simulink model "bitcrusher"  (R2020b)
settings: Solver=FixedStepDiscrete  StartTime=0.0  StopTime=stopTime  RelTol=1e-3
InitFcn:
  | initCallback
StopFcn:
  | stopCallback
values from neighbouring files (symbols this model uses):
  mp = sm_init_avalon_signals(mp)    [sm_callback_init.m]
settings Model: Creator=Ross  LastModifiedBy=wickh
settings DataIOCC: ReturnWorkspaceOutputs=off
settings OptimizationCC: BlockReduction=off  ConditionallyExecuteInputs=off  DefaultParameterBehavior=Inlined
settings DebuggingCC: ReadBeforeWriteMsg=DisableAll  WriteAfterWriteMsg=DisableAll  WriteAfterReadMsg=DisableAll  AlgebraicLoopMsg=error  MultiTaskDSMMsg=none  SingleTaskRateTransMsg=error  PregeneratedLibrarySubsystemCodeDiagnostic=none  ArithmeticOperatorsInVariantConditions=warning
settings HardwareCC: ProdBitPerPointer=32  ProdBitPerSizeT=32  ProdBitPerPtrDiffT=32  ProdLargestAtomicFloat=None  ProdIntDivRoundTo=Undefined  ProdEndianess=Unspecified  ProdWordSize=32  ProdHWDeviceType=ASIC/FPGA->ASIC/FPGA  TargetBitPerPointer=64  TargetBitPerSizeT=64  TargetBitPerPtrDiffT=64  TargetLongLongMode=on  TargetIntDivRoundTo=Zero  TargetEndianess=LittleEndian  TargetWordSize=64  TargetHWDeviceType=Custom Processor->MATLAB Host Computer  ProdEqTarget=off
settings ModelReferenceCC: UpdateModelReferenceTargets=IfOutOfDate
settings SFSimCC: SFSimEcho=off  SimUseLocalCustomCode=off  CustomCodeUndefinedFunction=UseInterfaceOnly
settings RTWCC: RTWUseLocalCustomCode=off

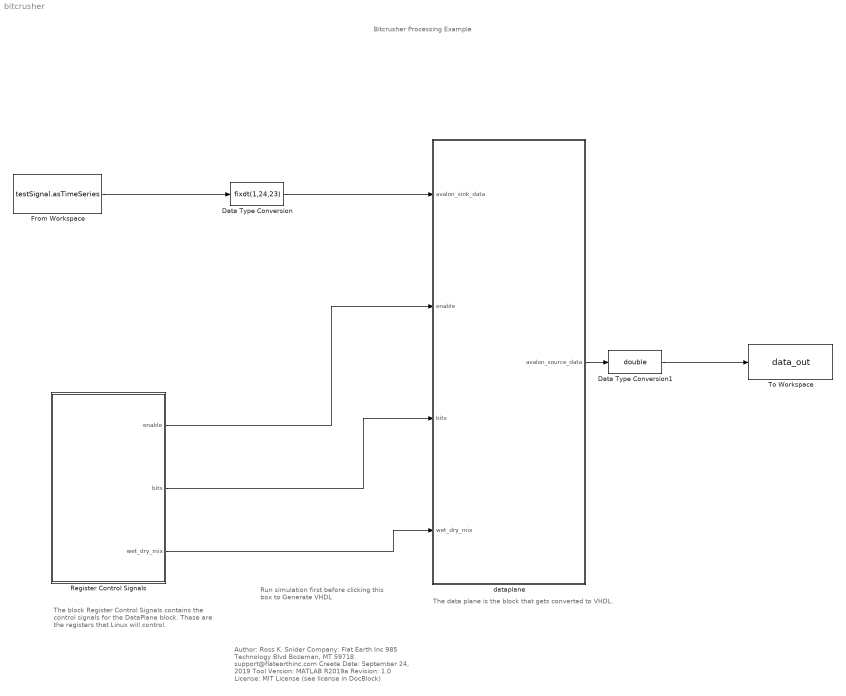
== system bitcrusher ==
  note: The data plane is the block that gets converted to VHDL.
  note: Author:          Ross K. Snider
      | Company:     Flat Earth Inc
      |                       985 Technology Blvd
      |                       Bozeman, MT 59718
      |                       support@flatearthinc.com
      | Create Date:  September 24, 2019
      | Tool Version:  MATLAB R2019a
      | Revision:        1.0
      | License:          MIT License (see license in DocBlock)
  note: Bitcrusher
      | Processing Example
  note: Run simulation first
      | before clicking this box to
      | Generate VHDL
  note: The block Register Control Signals contains
      | the control signals for the DataPlane block.
      | These are the registers that Linux will control.
  Data Type Conversion : DataTypeConversion  OutDataTypeStr=fixdt(1,24,23)
  Data Type Conversion1 : DataTypeConversion  OutDataTypeStr=double
  From Workspace : FromWorkspace  VariableName=testSignal.asTimeSeries  OutDataTypeStr=double  SampleTime=mp.Ts_sim  Interpolate=off  OutputAfterFinalValue=Setting to zero
  Register Control Signals : Subsystem
  To Workspace : ToWorkspace  VariableName=data_out  SampleTime=-1
  dataplane : Subsystem  TreatAsAtomicUnit=on
  wires:
  Data Type Conversion/1 -> dataplane/1(avalon_sink_data)
  Register Control Signals/2(bits) -> dataplane/3(bits)
  Register Control Signals/1(enable) -> dataplane/2(enable)
  Register Control Signals/3(wet_dry_mix) -> dataplane/4(wet_dry_mix)
  From Workspace/1 -> Data Type Conversion/1
  Data Type Conversion1/1 -> To Workspace/1
  dataplane/1(avalon_source_data) -> Data Type Conversion1/1

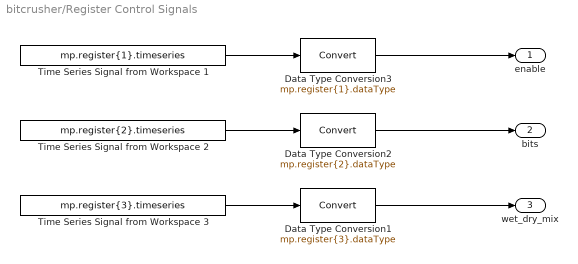
== system bitcrusher/Register Control Signals ==
  Data Type Conversion1 : DataTypeConversion  OutDataTypeStr=mp.register{3}.dataType
  Data Type Conversion2 : DataTypeConversion  OutDataTypeStr=mp.register{2}.dataType
  Data Type Conversion3 : DataTypeConversion  OutDataTypeStr=mp.register{1}.dataType
  Time Series Signal from Workspace 1 : FromWorkspace  VariableName=mp.register{1}.timeseries  OutDataTypeStr=double  SampleTime=mp.Ts_sim
  Time Series Signal from Workspace 2 : FromWorkspace  VariableName=mp.register{2}.timeseries  OutDataTypeStr=double  SampleTime=mp.Ts_sim
  Time Series Signal from Workspace 3 : FromWorkspace  VariableName=mp.register{3}.timeseries  OutDataTypeStr=double  SampleTime=mp.Ts_sim
  enable : Outport  VectorParamsAs1DForOutWhenUnconnected=off
  bits : Outport  Port=2  VectorParamsAs1DForOutWhenUnconnected=off
  wet_dry_mix : Outport  Port=3  VectorParamsAs1DForOutWhenUnconnected=off
  wires:
  Time Series Signal from Workspace 2/1 -> Data Type Conversion2/1
  Data Type Conversion2/1 -> bits/1
  Time Series Signal from Workspace 1/1 -> Data Type Conversion3/1
  Data Type Conversion3/1 -> enable/1
  Time Series Signal from Workspace 3/1 -> Data Type Conversion1/1
  Data Type Conversion1/1 -> wet_dry_mix/1

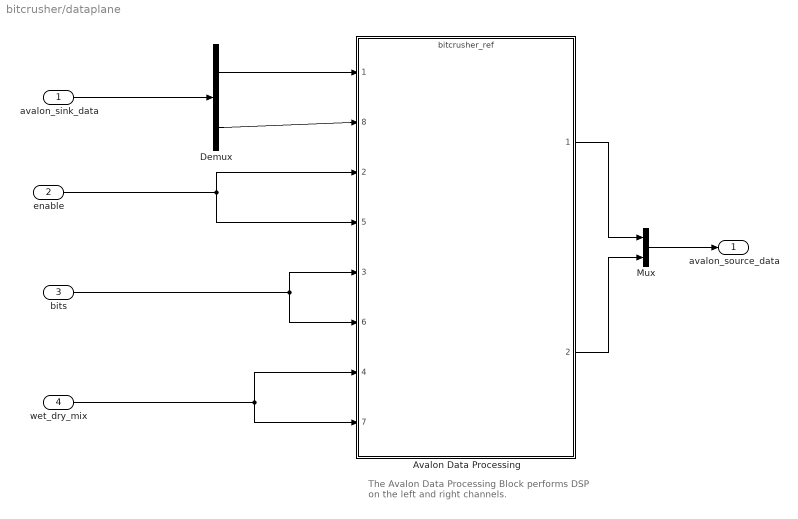
== system bitcrusher/dataplane ==
  note: The Avalon Data Processing Block
      | performs DSP on the left and right channels.
  avalon_sink_data : Inport
  enable : Inport  Port=2
  bits : Inport  Port=3
  wet_dry_mix : Inport  Port=4
  Avalon Data Processing : ModelReference  ModelNameDialog=bitcrusher_ref  SimulationMode=Normal  ModelReferenceVersion=3.10
      settings: PortSchema="{\"entries\":[{\"content\":{\"sides\":[{\"content\":{\"connectorIds\":[\"In1\",\"In8\",\"In2\",\"In5\",\"In3\",\"In6\",\"In4\",\"In7\"]},\"type\":\"ConnectorPlacement.EquallySpacedRectSide\",\"uuid\":\"cfc9476e-c101-4a90-ba08-effa479a8c46\"},{\"content\":{\"connectorIds\":[\"Out1\",\"Out2\"],\"side\":\"RIGHT\"},\"type\":\"ConnectorPlacement.EquallySpacedRectSide\",\"uuid\":\"4efa5dd5-d427-488d-bbaa-11ad48f52db2\"},{\"content\":{\"connectorIds\":[],\"side\":\"TOP\"},\"type\":\"ConnectorPlacement.EquallySpacedRectSide\",\"uuid\":\"d7e65a11-17aa-4e5c-94c4-a706f18cbe28\"},{\"content\":{\"connectorIds\":[],\"side\":\"HIDDEN\"},\"type\":\"ConnectorPlacement.EquallySpacedRectSide\",\"uuid\":\"578b30b2-4a86-4a40-9d9d-3e590ffd0d37\"}]},\"type\":\"ConnectorPlacement.EquallySpacedConnector\",\"uuid\":\"89dd9d33-f79f-4d92-a8dd-083ffe0e2010\"}],\"packageUris\":[\"http://schema.mathworks.com/mf0/Connector/R2020b\"],\"version\":\"1.0\"}"
  Demux : Demux  Outputs=2
  Mux : Mux  Inputs=2
  avalon_source_data : Outport  VectorParamsAs1DForOutWhenUnconnected=off
  wires:
  bits/1 -> Avalon Data Processing/3, Avalon Data Processing/6
  enable/1 -> Avalon Data Processing/2, Avalon Data Processing/5
  wet_dry_mix/1 -> Avalon Data Processing/4, Avalon Data Processing/7
  Demux/1 -> Avalon Data Processing/1
  Demux/2 -> Avalon Data Processing/8
  avalon_sink_data/1 -> Demux/1
  Avalon Data Processing/1 -> Mux/1
  Avalon Data Processing/2 -> Mux/2
  Mux/1 -> avalon_source_data/1
